simulink model "SRM_IOT"  (R2024b)
settings: Solver=VariableStepAuto  StartTime=0.0  StopTime=10.0  RelTol=1e-3
undefined symbols (not defined in the file): Ion, Lithium, sigbuilder_block
libraries: spsBreakerLib x120, spsSeriesRLCBranchLib x70, spsBatteryLib x42, spsIdealSwitchLib x33, spsVoltageMeasurementLib x27, slpidlib x17, spsMosfetLib x17, spsPWMGeneratorDCDCLib x11, spsDiodeLib x6, spsCurrentMeasurementLib x4, spsIGBTLib x2, spsThreePhaseSeriesRLCLoadLib x2
(part 3 of 5)

== system SRM_IOT/Subsystem18/Subsystem4 ==
  Battery : spsBatteryLib/Battery  BatType=Lithium-Ion  NomV=12  NomQ=10  SOC=95  Batt_Tr=30  PresetModel=on  MaxQ=10  MinV=9  FullV=13.9678  Dis_rate=4.3478  R=0.012  Normal_OP=9.0435  expZone="[12.9646     0.491304]"
  Breaker{,1..3} (4 alike) : spsBreakerLib/Breaker  InitialState=0  SwitchingTimes="[1/60  5/60]"  External=on  BreakerResistance=0.01  SnubberResistance=1e6  SnubberCapacitance=inf  Measurements=None  MoreParameters=on  NoBreakLoop=off
  Bus Selector : BusSelector  OutputSignals=SOC (%),Current (A),Voltage (V)
  Scope : Scope  NumInputPorts=3
  Series RLC Branch : spsSeriesRLCBranchLib/Series RLC Branch  LConnTagsString=__new0  RConnTagsString=__new0  BranchType=R  Resistance=1  Inductance=1e-3  SetiL0=off  InitialCurrent=0  Capacitance=1e-6  Setx0=off  InitialVoltage=0  Measurements=None
  + : PMIOPort  Side=Right
  - : PMIOPort  Port=2  Side=Right
  tag scope: s3=global
  wires:
  Battery/1 -> Bus Selector/1
  [c3] -> Breaker3/1, Breaker/1
  Bus Selector/2 -> Scope/2  "<Current (A)>"
  [d3] -> Breaker1/1, Breaker2/1
  Bus Selector/3 -> Scope/3  "<Voltage (V)>"
  Bus Selector/1 -> [s3], Scope/1  "<SOC (%)>"
  connections:
  Breaker2/LConn1 -- Breaker3/RConn1 -- Battery/LConn2
  Breaker1/LConn1 -- Battery/LConn1 -- Breaker/RConn1
  +/RConn1 -- Breaker/LConn1
  Series RLC Branch/LConn1 -- Breaker2/RConn1
  Series RLC Branch/RConn1 -- Breaker1/RConn1
  -/RConn1 -- Breaker3/LConn1

== system SRM_IOT/Subsystem18/Subsystem5 ==
  Battery : spsBatteryLib/Battery  BatType=Lithium-Ion  NomV=12  NomQ=10  SOC=95  Batt_Tr=30  PresetModel=on  MaxQ=10  MinV=9  FullV=13.9678  Dis_rate=4.3478  R=0.012  Normal_OP=9.0435  expZone="[12.9646     0.491304]"
  Breaker{,1..3} (4 alike) : spsBreakerLib/Breaker  InitialState=0  SwitchingTimes="[1/60  5/60]"  External=on  BreakerResistance=0.01  SnubberResistance=1e6  SnubberCapacitance=inf  Measurements=None  MoreParameters=on  NoBreakLoop=off
  Bus Selector : BusSelector  OutputSignals=SOC (%),Current (A),Voltage (V)
  Scope : Scope  NumInputPorts=3
  Series RLC Branch : spsSeriesRLCBranchLib/Series RLC Branch  LConnTagsString=__new0  RConnTagsString=__new0  BranchType=R  Resistance=1  Inductance=1e-3  SetiL0=off  InitialCurrent=0  Capacitance=1e-6  Setx0=off  InitialVoltage=0  Measurements=None
  + : PMIOPort  Side=Right
  - : PMIOPort  Port=2  Side=Right
  tag scope: s2=global
  wires:
  Battery/1 -> Bus Selector/1
  [c2] -> Breaker3/1, Breaker/1
  Bus Selector/2 -> Scope/2  "<Current (A)>"
  [d2] -> Breaker1/1, Breaker2/1
  Bus Selector/3 -> Scope/3  "<Voltage (V)>"
  Bus Selector/1 -> [s2], Scope/1  "<SOC (%)>"
  connections:
  Breaker2/LConn1 -- Breaker3/RConn1 -- Battery/LConn2
  Breaker1/LConn1 -- Battery/LConn1 -- Breaker/RConn1
  +/RConn1 -- Breaker/LConn1
  Series RLC Branch/LConn1 -- Breaker2/RConn1
  Series RLC Branch/RConn1 -- Breaker1/RConn1
  -/RConn1 -- Breaker3/LConn1

== system SRM_IOT/Subsystem18/Subsystem6 ==
  Battery : spsBatteryLib/Battery  BatType=Lithium-Ion  NomV=12  NomQ=10  SOC=95  Batt_Tr=30  PresetModel=on  MaxQ=10  MinV=9  FullV=13.9678  Dis_rate=4.3478  R=0.012  Normal_OP=9.0435  expZone="[12.9646     0.491304]"
  Breaker{,1..3} (4 alike) : spsBreakerLib/Breaker  InitialState=0  SwitchingTimes="[1/60  5/60]"  External=on  BreakerResistance=0.01  SnubberResistance=1e6  SnubberCapacitance=inf  Measurements=None  MoreParameters=on  NoBreakLoop=off
  Bus Selector : BusSelector  OutputSignals=SOC (%),Current (A),Voltage (V)
  Scope : Scope  NumInputPorts=3
  Series RLC Branch : spsSeriesRLCBranchLib/Series RLC Branch  LConnTagsString=__new0  RConnTagsString=__new0  BranchType=R  Resistance=1  Inductance=1e-3  SetiL0=off  InitialCurrent=0  Capacitance=1e-6  Setx0=off  InitialVoltage=0  Measurements=None
  + : PMIOPort  Side=Right
  - : PMIOPort  Port=2  Side=Right
  tag scope: s15=global
  wires:
  Battery/1 -> Bus Selector/1
  [c15] -> Breaker3/1, Breaker/1
  Bus Selector/2 -> Scope/2  "<Current (A)>"
  [d15] -> Breaker1/1, Breaker2/1
  Bus Selector/3 -> Scope/3  "<Voltage (V)>"
  Bus Selector/1 -> [s15], Scope/1  "<SOC (%)>"
  connections:
  Breaker2/LConn1 -- Breaker3/RConn1 -- Battery/LConn2
  Breaker1/LConn1 -- Battery/LConn1 -- Breaker/RConn1
  +/RConn1 -- Breaker/LConn1
  Series RLC Branch/LConn1 -- Breaker2/RConn1
  Series RLC Branch/RConn1 -- Breaker1/RConn1
  -/RConn1 -- Breaker3/LConn1

== system SRM_IOT/Subsystem18/Subsystem7 ==
  Battery : spsBatteryLib/Battery  BatType=Lithium-Ion  NomV=12  NomQ=10  SOC=95  Batt_Tr=30  PresetModel=on  MaxQ=10  MinV=9  FullV=13.9678  Dis_rate=4.3478  R=0.012  Normal_OP=9.0435  expZone="[12.9646     0.491304]"
  Breaker{,1..3} (4 alike) : spsBreakerLib/Breaker  InitialState=0  SwitchingTimes="[1/60  5/60]"  External=on  BreakerResistance=0.01  SnubberResistance=1e6  SnubberCapacitance=inf  Measurements=None  MoreParameters=on  NoBreakLoop=off
  Bus Selector : BusSelector  OutputSignals=SOC (%),Current (A),Voltage (V)
  Scope : Scope  NumInputPorts=3
  Series RLC Branch : spsSeriesRLCBranchLib/Series RLC Branch  LConnTagsString=__new0  RConnTagsString=__new0  BranchType=R  Resistance=1  Inductance=1e-3  SetiL0=off  InitialCurrent=0  Capacitance=1e-6  Setx0=off  InitialVoltage=0  Measurements=None
  + : PMIOPort  Side=Right
  - : PMIOPort  Port=2  Side=Right
  tag scope: s11=global
  wires:
  Battery/1 -> Bus Selector/1
  [c11] -> Breaker3/1, Breaker/1
  Bus Selector/2 -> Scope/2  "<Current (A)>"
  [d11] -> Breaker1/1, Breaker2/1
  Bus Selector/3 -> Scope/3  "<Voltage (V)>"
  Bus Selector/1 -> [s11], Scope/1  "<SOC (%)>"
  connections:
  Breaker2/LConn1 -- Breaker3/RConn1 -- Battery/LConn2
  Breaker1/LConn1 -- Battery/LConn1 -- Breaker/RConn1
  +/RConn1 -- Breaker/LConn1
  Series RLC Branch/LConn1 -- Breaker2/RConn1
  Series RLC Branch/RConn1 -- Breaker1/RConn1
  -/RConn1 -- Breaker3/LConn1

== system SRM_IOT/Subsystem18/Subsystem8 ==
  Battery : spsBatteryLib/Battery  BatType=Lithium-Ion  NomV=12  NomQ=10  SOC=95  Batt_Tr=30  PresetModel=on  MaxQ=10  MinV=9  FullV=13.9678  Dis_rate=4.3478  R=0.012  Normal_OP=9.0435  expZone="[12.9646     0.491304]"
  Breaker{,1..3} (4 alike) : spsBreakerLib/Breaker  InitialState=0  SwitchingTimes="[1/60  5/60]"  External=on  BreakerResistance=0.01  SnubberResistance=1e6  SnubberCapacitance=inf  Measurements=None  MoreParameters=on  NoBreakLoop=off
  Bus Selector : BusSelector  OutputSignals=SOC (%),Current (A),Voltage (V)
  Scope : Scope  NumInputPorts=3
  Series RLC Branch : spsSeriesRLCBranchLib/Series RLC Branch  LConnTagsString=__new0  RConnTagsString=__new0  BranchType=R  Resistance=1  Inductance=1e-3  SetiL0=off  InitialCurrent=0  Capacitance=1e-6  Setx0=off  InitialVoltage=0  Measurements=None
  + : PMIOPort  Side=Right
  - : PMIOPort  Port=2  Side=Right
  tag scope: s19=global
  wires:
  Battery/1 -> Bus Selector/1
  [c19] -> Breaker3/1, Breaker/1
  Bus Selector/2 -> Scope/2  "<Current (A)>"
  [d19] -> Breaker1/1, Breaker2/1
  Bus Selector/3 -> Scope/3  "<Voltage (V)>"
  Bus Selector/1 -> [s19], Scope/1  "<SOC (%)>"
  connections:
  Breaker2/LConn1 -- Breaker3/RConn1 -- Battery/LConn2
  Breaker1/LConn1 -- Battery/LConn1 -- Breaker/RConn1
  +/RConn1 -- Breaker/LConn1
  Series RLC Branch/LConn1 -- Breaker2/RConn1
  Series RLC Branch/RConn1 -- Breaker1/RConn1
  -/RConn1 -- Breaker3/LConn1

== system SRM_IOT/Subsystem18/Subsystem9 ==
  Battery : spsBatteryLib/Battery  BatType=Lithium-Ion  NomV=12  NomQ=10  SOC=95  Batt_Tr=30  PresetModel=on  MaxQ=10  MinV=9  FullV=13.9678  Dis_rate=4.3478  R=0.012  Normal_OP=9.0435  expZone="[12.9646     0.491304]"
  Breaker{,1..3} (4 alike) : spsBreakerLib/Breaker  InitialState=0  SwitchingTimes="[1/60  5/60]"  External=on  BreakerResistance=0.01  SnubberResistance=1e6  SnubberCapacitance=inf  Measurements=None  MoreParameters=on  NoBreakLoop=off
  Bus Selector : BusSelector  OutputSignals=SOC (%),Current (A),Voltage (V)
  Scope : Scope  NumInputPorts=3
  Series RLC Branch : spsSeriesRLCBranchLib/Series RLC Branch  LConnTagsString=__new0  RConnTagsString=__new0  BranchType=R  Resistance=1  Inductance=1e-3  SetiL0=off  InitialCurrent=0  Capacitance=1e-6  Setx0=off  InitialVoltage=0  Measurements=None
  + : PMIOPort  Side=Right
  - : PMIOPort  Port=2  Side=Right
  tag scope: s20=global
  wires:
  Battery/1 -> Bus Selector/1
  [c20] -> Breaker3/1, Breaker/1
  Bus Selector/2 -> Scope/2  "<Current (A)>"
  [d20] -> Breaker1/1, Breaker2/1
  Bus Selector/3 -> Scope/3  "<Voltage (V)>"
  Bus Selector/1 -> [s20], Scope/1  "<SOC (%)>"
  connections:
  Breaker2/LConn1 -- Breaker3/RConn1 -- Battery/LConn2
  Breaker1/LConn1 -- Battery/LConn1 -- Breaker/RConn1
  +/RConn1 -- Breaker/LConn1
  Series RLC Branch/LConn1 -- Breaker2/RConn1
  Series RLC Branch/RConn1 -- Breaker1/RConn1
  -/RConn1 -- Breaker3/LConn1

== system SRM_IOT/Subsystem2/Control ==
  Add : Sum  Inputs=+-
  Add1 : Sum  Inputs=+-
  Constant : Constant  Value=25.99
  Gain : Gain  Gain=-1
  NOT : Logic  Operator=NOT  IconShape=distinctive  AllPortsSameDT=off  OutDataTypeStr=boolean
  PID Controller : slpidlib/PID Controller  Controller=PI  Form=Parallel  TimeDomain=Continuous-time  UseExternalTs=off  SampleTime=-1  IntegratorMethod=Forward Euler  FilterMethod=Forward Euler  ControllerParametersSource=internal  P=0.005  I=10  UseKiTs=off  D=0  UseExternalDerivativeSource=off  N=100  UseFilter=on  TunerSelectOption=Transfer Function Based (PID Tuner App)  InitialConditionSource=internal  InitialConditionForIntegrator=0.54  InitialConditionForFilter=0  DifferentiatorICPrevScaledInput=0  ExternalReset=none  TrackingMode=off  Kt=1  LimitOutput=on  SatLimitsSource=internal  UpperSaturationLimit=0.975  LowerSaturationLimit=0  LinearizeAsGain=on  AntiWindupMode=none  Kb=1  LimitIntegrator=off  UpperIntegratorSaturationLimit=inf  LowerIntegratorSaturationLimit=-inf  POutMin=[]  POutMax=[]  IOutMin=[]  IOutMax=[]  DOutMin=[]  DOutMax=[]  NOutMin=[]  NOutMax=[]  SumOutMin=[]  SumOutMax=[]  SaturationOutMin=[]  SaturationOutMax=[]  PParamMin=[]  PParamMax=[]  IParamMin=[]  IParamMax=[]  DParamMin=[]  DParamMax=[]  NParamMin=[]  NParamMax=[]  KbParamMin=[]  KbParamMax=[]  KtParamMin=[]  KtParamMax=[]  KbOutMin=[]  KbOutMax=[]  KtOutMin=[]  KtOutMax=[]  IntegratorOutMin=[]  IntegratorOutMax=[]  FilterOutMin=[]  FilterOutMax=[]  SumI1OutMin=[]  SumI1OutMax=[]  SumI2OutMin=[]  SumI2OutMax=[]  SumI3OutMin=[]  SumI3OutMax=[]  SumI4OutMin=[]  SumI4OutMax=[]  SumDOutMin=[]  SumDOutMax=[]  DifferentiatorOutMin=[]  DifferentiatorOutMax=[]  FilterDiffOutCoefMin=[]  FilterDiffOutCoefMax=[]  ReciprocalOutMin=[]  ReciprocalOutMax=[]  SumDenOutMin=[]  SumDenOutMax=[]  SumNumOutMin=[]  SumNumOutMax=[]  DivideOutMin=[]  DivideOutMax=[]  UdiffTsProdOutMin=[]  UdiffTsProdOutMax=[]  NTsProdOutMin=[]  NTsProdOutMax=[]  UintegralTsProdOutMin=[]  UintegralTsProdOutMax=[]  UngainTsProdOutMin=[]  UngainTsProdOutMax=[]  ClampingZeroOutDataTypeStr=Inherit: Inherit via back propagation  ClampingZeroOutMin=[]  ClampingZeroOutMax=[]  FilterDenConstantOutDataTypeStr=Inherit: Inherit via back propagation  FilterDenConstantOutMin=[]  FilterDenConstantOutMax=[]  PCopyOutDataTypeStr=Inherit: Inherit via back propagation  PCopyOutMin=[]  PCopyOutMax=[]  NCopyOutDataTypeStr=Inherit: Inherit via back propagation  NCopyOutMin=[]  NCopyOutMax=[]  IntegratorContinuousStateAttributes=''  IntegratorStateMustResolveToSignalObject=off  IntegratorRTWStateStorageClass=Auto  FilterContinuousStateAttributes=''  FilterStateMustResolveToSignalObject=off  FilterRTWStateStorageClass=Auto  ParallelPVariant=InternalParameters  IdealPVariant=Disabled  IVariant=InternalParameters  DVariant=Disabled  IntegratorVariant=Continuous  SatVariant=Enabled  AWVariant=Passthrough  PCopyVariant=Disabled  TRVariant=Disabled  FdbkBlocksVariant=Forward  IdealPFdbkVariant=Disabled  SatFdbkVariant=Disabled  DerivativeFilterVariant=Disabled  NVariant=Disabled  NCopyVariant=Disabled_SignalSpec  FilterICVariant=Disabled  IntegratorICVariant=InternalICs  ExternalResetVariant=Disabled  TRSumVariant=Passthrough  SumFdbkVariant=Disabled  SumVariant=Sum_PI  TsampFilterVariant=InternalTs  TsampNgainVariant=Passthrough  TsampIntegralVariant=Disabled_SignalSpec  ExternalSaturationOutDataTypeStr=Inherit: Same as second input  DerivativeSourceVariant=Disabled  PreIntVariant=InternalPreInt
  PID Controller1 : slpidlib/PID Controller  Controller=PI  Form=Parallel  TimeDomain=Continuous-time  UseExternalTs=off  SampleTime=-1  IntegratorMethod=Forward Euler  FilterMethod=Forward Euler  ControllerParametersSource=internal  P=40  I=2000  UseKiTs=off  D=0  UseExternalDerivativeSource=off  N=100  UseFilter=on  TunerSelectOption=Transfer Function Based (PID Tuner App)  InitialConditionSource=internal  InitialConditionForIntegrator=0.54  InitialConditionForFilter=0  DifferentiatorICPrevScaledInput=0  ExternalReset=none  TrackingMode=off  Kt=1  LimitOutput=on  SatLimitsSource=internal  UpperSaturationLimit=17.39  LowerSaturationLimit=0  LinearizeAsGain=on  AntiWindupMode=none  Kb=1  LimitIntegrator=off  UpperIntegratorSaturationLimit=inf  LowerIntegratorSaturationLimit=-inf  POutMin=[]  POutMax=[]  IOutMin=[]  IOutMax=[]  DOutMin=[]  DOutMax=[]  NOutMin=[]  NOutMax=[]  SumOutMin=[]  SumOutMax=[]  SaturationOutMin=[]  SaturationOutMax=[]  PParamMin=[]  PParamMax=[]  IParamMin=[]  IParamMax=[]  DParamMin=[]  DParamMax=[]  NParamMin=[]  NParamMax=[]  KbParamMin=[]  KbParamMax=[]  KtParamMin=[]  KtParamMax=[]  KbOutMin=[]  KbOutMax=[]  KtOutMin=[]  KtOutMax=[]  IntegratorOutMin=[]  IntegratorOutMax=[]  FilterOutMin=[]  FilterOutMax=[]  SumI1OutMin=[]  SumI1OutMax=[]  SumI2OutMin=[]  SumI2OutMax=[]  SumI3OutMin=[]  SumI3OutMax=[]  SumI4OutMin=[]  SumI4OutMax=[]  SumDOutMin=[]  SumDOutMax=[]  DifferentiatorOutMin=[]  DifferentiatorOutMax=[]  FilterDiffOutCoefMin=[]  FilterDiffOutCoefMax=[]  ReciprocalOutMin=[]  ReciprocalOutMax=[]  SumDenOutMin=[]  SumDenOutMax=[]  SumNumOutMin=[]  SumNumOutMax=[]  DivideOutMin=[]  DivideOutMax=[]  UdiffTsProdOutMin=[]  UdiffTsProdOutMax=[]  NTsProdOutMin=[]  NTsProdOutMax=[]  UintegralTsProdOutMin=[]  UintegralTsProdOutMax=[]  UngainTsProdOutMin=[]  UngainTsProdOutMax=[]  ClampingZeroOutDataTypeStr=Inherit: Inherit via back propagation  ClampingZeroOutMin=[]  ClampingZeroOutMax=[]  FilterDenConstantOutDataTypeStr=Inherit: Inherit via back propagation  FilterDenConstantOutMin=[]  FilterDenConstantOutMax=[]  PCopyOutDataTypeStr=Inherit: Inherit via back propagation  PCopyOutMin=[]  PCopyOutMax=[]  NCopyOutDataTypeStr=Inherit: Inherit via back propagation  NCopyOutMin=[]  NCopyOutMax=[]  IntegratorContinuousStateAttributes=''  IntegratorStateMustResolveToSignalObject=off  IntegratorRTWStateStorageClass=Auto  FilterContinuousStateAttributes=''  FilterStateMustResolveToSignalObject=off  FilterRTWStateStorageClass=Auto  ParallelPVariant=InternalParameters  IdealPVariant=Disabled  IVariant=InternalParameters  DVariant=Disabled  IntegratorVariant=Continuous  SatVariant=Enabled  AWVariant=Passthrough  PCopyVariant=Disabled  TRVariant=Disabled  FdbkBlocksVariant=Forward  IdealPFdbkVariant=Disabled  SatFdbkVariant=Disabled  DerivativeFilterVariant=Disabled  NVariant=Disabled  NCopyVariant=Disabled_SignalSpec  FilterICVariant=Disabled  IntegratorICVariant=InternalICs  ExternalResetVariant=Disabled  TRSumVariant=Passthrough  SumFdbkVariant=Disabled  SumVariant=Sum_PI  TsampFilterVariant=InternalTs  TsampNgainVariant=Passthrough  TsampIntegralVariant=Disabled_SignalSpec  ExternalSaturationOutDataTypeStr=Inherit: Same as second input  DerivativeSourceVariant=Disabled  PreIntVariant=InternalPreInt
  PWM Generator (DC-DC) : spsPWMGeneratorDCDCLib/PWM Generator (DC-DC)  Fsw=10e3  Ts=5e-6
  tag scope: Mosfet_333=global, Mosfet_33=global
  wires:
  Add/1 -> PID Controller/1
  PWM Generator (DC-DC)/1 -> NOT/1, [Mosfet_33]
  PID Controller/1 -> PWM Generator (DC-DC)/1
  NOT/1 -> [Mosfet_333]
  [Ref_Current] -> Add/2
  [Current] -> Add/1
  PID Controller1/1 -> Gain/1
  Gain/1 -> [Ref_Current]
  Add1/1 -> PID Controller1/1
  Constant/1 -> Add1/1
  [Voltage] -> Add1/2

== system SRM_IOT/Subsystem3/Control ==
  Add : Sum  Inputs=+-
  Add1 : Sum  Inputs=+-
  Constant : Constant  Value=25.99
  Gain : Gain  Gain=-1
  NOT : Logic  Operator=NOT  IconShape=distinctive  AllPortsSameDT=off  OutDataTypeStr=boolean
  PID Controller : slpidlib/PID Controller  Controller=PI  Form=Parallel  TimeDomain=Continuous-time  UseExternalTs=off  SampleTime=-1  IntegratorMethod=Forward Euler  FilterMethod=Forward Euler  ControllerParametersSource=internal  P=0.005  I=10  UseKiTs=off  D=0  UseExternalDerivativeSource=off  N=100  UseFilter=on  TunerSelectOption=Transfer Function Based (PID Tuner App)  InitialConditionSource=internal  InitialConditionForIntegrator=0.54  InitialConditionForFilter=0  DifferentiatorICPrevScaledInput=0  ExternalReset=none  TrackingMode=off  Kt=1  LimitOutput=on  SatLimitsSource=internal  UpperSaturationLimit=0.975  LowerSaturationLimit=0  LinearizeAsGain=on  AntiWindupMode=none  Kb=1  LimitIntegrator=off  UpperIntegratorSaturationLimit=inf  LowerIntegratorSaturationLimit=-inf  POutMin=[]  POutMax=[]  IOutMin=[]  IOutMax=[]  DOutMin=[]  DOutMax=[]  NOutMin=[]  NOutMax=[]  SumOutMin=[]  SumOutMax=[]  SaturationOutMin=[]  SaturationOutMax=[]  PParamMin=[]  PParamMax=[]  IParamMin=[]  IParamMax=[]  DParamMin=[]  DParamMax=[]  NParamMin=[]  NParamMax=[]  KbParamMin=[]  KbParamMax=[]  KtParamMin=[]  KtParamMax=[]  KbOutMin=[]  KbOutMax=[]  KtOutMin=[]  KtOutMax=[]  IntegratorOutMin=[]  IntegratorOutMax=[]  FilterOutMin=[]  FilterOutMax=[]  SumI1OutMin=[]  SumI1OutMax=[]  SumI2OutMin=[]  SumI2OutMax=[]  SumI3OutMin=[]  SumI3OutMax=[]  SumI4OutMin=[]  SumI4OutMax=[]  SumDOutMin=[]  SumDOutMax=[]  DifferentiatorOutMin=[]  DifferentiatorOutMax=[]  FilterDiffOutCoefMin=[]  FilterDiffOutCoefMax=[]  ReciprocalOutMin=[]  ReciprocalOutMax=[]  SumDenOutMin=[]  SumDenOutMax=[]  SumNumOutMin=[]  SumNumOutMax=[]  DivideOutMin=[]  DivideOutMax=[]  UdiffTsProdOutMin=[]  UdiffTsProdOutMax=[]  NTsProdOutMin=[]  NTsProdOutMax=[]  UintegralTsProdOutMin=[]  UintegralTsProdOutMax=[]  UngainTsProdOutMin=[]  UngainTsProdOutMax=[]  ClampingZeroOutDataTypeStr=Inherit: Inherit via back propagation  ClampingZeroOutMin=[]  ClampingZeroOutMax=[]  FilterDenConstantOutDataTypeStr=Inherit: Inherit via back propagation  FilterDenConstantOutMin=[]  FilterDenConstantOutMax=[]  PCopyOutDataTypeStr=Inherit: Inherit via back propagation  PCopyOutMin=[]  PCopyOutMax=[]  NCopyOutDataTypeStr=Inherit: Inherit via back propagation  NCopyOutMin=[]  NCopyOutMax=[]  IntegratorContinuousStateAttributes=''  IntegratorStateMustResolveToSignalObject=off  IntegratorRTWStateStorageClass=Auto  FilterContinuousStateAttributes=''  FilterStateMustResolveToSignalObject=off  FilterRTWStateStorageClass=Auto  ParallelPVariant=InternalParameters  IdealPVariant=Disabled  IVariant=InternalParameters  DVariant=Disabled  IntegratorVariant=Continuous  SatVariant=Enabled  AWVariant=Passthrough  PCopyVariant=Disabled  TRVariant=Disabled  FdbkBlocksVariant=Forward  IdealPFdbkVariant=Disabled  SatFdbkVariant=Disabled  DerivativeFilterVariant=Disabled  NVariant=Disabled  NCopyVariant=Disabled_SignalSpec  FilterICVariant=Disabled  IntegratorICVariant=InternalICs  ExternalResetVariant=Disabled  TRSumVariant=Passthrough  SumFdbkVariant=Disabled  SumVariant=Sum_PI  TsampFilterVariant=InternalTs  TsampNgainVariant=Passthrough  TsampIntegralVariant=Disabled_SignalSpec  ExternalSaturationOutDataTypeStr=Inherit: Same as second input  DerivativeSourceVariant=Disabled  PreIntVariant=InternalPreInt
  PID Controller1 : slpidlib/PID Controller  Controller=PI  Form=Parallel  TimeDomain=Continuous-time  UseExternalTs=off  SampleTime=-1  IntegratorMethod=Forward Euler  FilterMethod=Forward Euler  ControllerParametersSource=internal  P=40  I=2000  UseKiTs=off  D=0  UseExternalDerivativeSource=off  N=100  UseFilter=on  TunerSelectOption=Transfer Function Based (PID Tuner App)  InitialConditionSource=internal  InitialConditionForIntegrator=0.54  InitialConditionForFilter=0  DifferentiatorICPrevScaledInput=0  ExternalReset=none  TrackingMode=off  Kt=1  LimitOutput=on  SatLimitsSource=internal  UpperSaturationLimit=17.39  LowerSaturationLimit=0  LinearizeAsGain=on  AntiWindupMode=none  Kb=1  LimitIntegrator=off  UpperIntegratorSaturationLimit=inf  LowerIntegratorSaturationLimit=-inf  POutMin=[]  POutMax=[]  IOutMin=[]  IOutMax=[]  DOutMin=[]  DOutMax=[]  NOutMin=[]  NOutMax=[]  SumOutMin=[]  SumOutMax=[]  SaturationOutMin=[]  SaturationOutMax=[]  PParamMin=[]  PParamMax=[]  IParamMin=[]  IParamMax=[]  DParamMin=[]  DParamMax=[]  NParamMin=[]  NParamMax=[]  KbParamMin=[]  KbParamMax=[]  KtParamMin=[]  KtParamMax=[]  KbOutMin=[]  KbOutMax=[]  KtOutMin=[]  KtOutMax=[]  IntegratorOutMin=[]  IntegratorOutMax=[]  FilterOutMin=[]  FilterOutMax=[]  SumI1OutMin=[]  SumI1OutMax=[]  SumI2OutMin=[]  SumI2OutMax=[]  SumI3OutMin=[]  SumI3OutMax=[]  SumI4OutMin=[]  SumI4OutMax=[]  SumDOutMin=[]  SumDOutMax=[]  DifferentiatorOutMin=[]  DifferentiatorOutMax=[]  FilterDiffOutCoefMin=[]  FilterDiffOutCoefMax=[]  ReciprocalOutMin=[]  ReciprocalOutMax=[]  SumDenOutMin=[]  SumDenOutMax=[]  SumNumOutMin=[]  SumNumOutMax=[]  DivideOutMin=[]  DivideOutMax=[]  UdiffTsProdOutMin=[]  UdiffTsProdOutMax=[]  NTsProdOutMin=[]  NTsProdOutMax=[]  UintegralTsProdOutMin=[]  UintegralTsProdOutMax=[]  UngainTsProdOutMin=[]  UngainTsProdOutMax=[]  ClampingZeroOutDataTypeStr=Inherit: Inherit via back propagation  ClampingZeroOutMin=[]  ClampingZeroOutMax=[]  FilterDenConstantOutDataTypeStr=Inherit: Inherit via back propagation  FilterDenConstantOutMin=[]  FilterDenConstantOutMax=[]  PCopyOutDataTypeStr=Inherit: Inherit via back propagation  PCopyOutMin=[]  PCopyOutMax=[]  NCopyOutDataTypeStr=Inherit: Inherit via back propagation  NCopyOutMin=[]  NCopyOutMax=[]  IntegratorContinuousStateAttributes=''  IntegratorStateMustResolveToSignalObject=off  IntegratorRTWStateStorageClass=Auto  FilterContinuousStateAttributes=''  FilterStateMustResolveToSignalObject=off  FilterRTWStateStorageClass=Auto  ParallelPVariant=InternalParameters  IdealPVariant=Disabled  IVariant=InternalParameters  DVariant=Disabled  IntegratorVariant=Continuous  SatVariant=Enabled  AWVariant=Passthrough  PCopyVariant=Disabled  TRVariant=Disabled  FdbkBlocksVariant=Forward  IdealPFdbkVariant=Disabled  SatFdbkVariant=Disabled  DerivativeFilterVariant=Disabled  NVariant=Disabled  NCopyVariant=Disabled_SignalSpec  FilterICVariant=Disabled  IntegratorICVariant=InternalICs  ExternalResetVariant=Disabled  TRSumVariant=Passthrough  SumFdbkVariant=Disabled  SumVariant=Sum_PI  TsampFilterVariant=InternalTs  TsampNgainVariant=Passthrough  TsampIntegralVariant=Disabled_SignalSpec  ExternalSaturationOutDataTypeStr=Inherit: Same as second input  DerivativeSourceVariant=Disabled  PreIntVariant=InternalPreInt
  PWM Generator (DC-DC) : spsPWMGeneratorDCDCLib/PWM Generator (DC-DC)  Fsw=10e3  Ts=5e-6
  tag scope: Mosfet_444=global, Mosfet_44=global
  wires:
  Add/1 -> PID Controller/1
  PWM Generator (DC-DC)/1 -> NOT/1, [Mosfet_44]
  PID Controller/1 -> PWM Generator (DC-DC)/1
  NOT/1 -> [Mosfet_444]
  [Ref_Current] -> Add/2
  [Current] -> Add/1
  PID Controller1/1 -> Gain/1
  Gain/1 -> [Ref_Current]
  Add1/1 -> PID Controller1/1
  Constant/1 -> Add1/1
  [Voltage] -> Add1/2

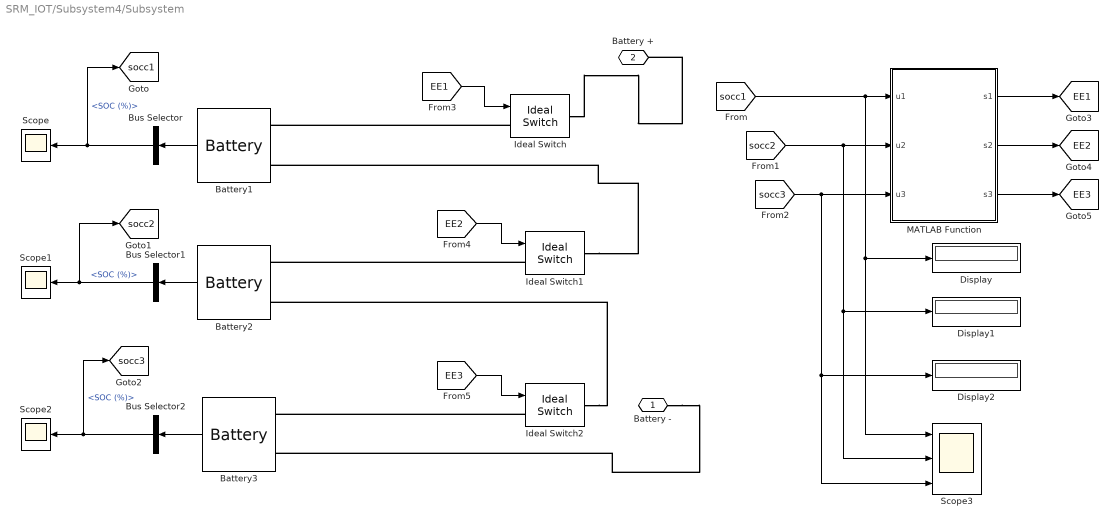
== system SRM_IOT/Subsystem4/Subsystem ==
  Battery1 : spsBatteryLib/Battery  BatType=Lithium-Ion  NomV=3.6  NomQ=4  SOC=100  Batt_Tr=1  PresetModel=on  MaxQ=4  MinV=2.7  FullV=4.1904  Dis_rate=1.7391  R=0.009  Normal_OP=3.6174  expZone="[3.8894     0.19652]"
  Battery2 : spsBatteryLib/Battery  BatType=Lithium-Ion  NomV=3.6  NomQ=4  SOC=60  Batt_Tr=1  PresetModel=on  MaxQ=4  MinV=2.7  FullV=4.1904  Dis_rate=1.7391  R=0.009  Normal_OP=3.6174  expZone="[3.8894     0.19652]"
  Battery3 : spsBatteryLib/Battery  BatType=Lithium-Ion  NomV=3.6  NomQ=4  SOC=30  Batt_Tr=1  PresetModel=on  MaxQ=4  MinV=2.7  FullV=4.1904  Dis_rate=1.7391  R=0.009  Normal_OP=3.6174  expZone="[3.8894     0.19652]"
  Bus Selector : BusSelector  OutputSignals=SOC (%)
  Bus Selector1 : BusSelector  OutputSignals=SOC (%)
  Bus Selector2 : BusSelector  OutputSignals=SOC (%)
  Display : Display
  Display1 : Display
  Display2 : Display
  Ideal Switch : spsIdealSwitchLib/Ideal Switch  Ron=0.001  Lon=0  IC=0  Rs=1e5  Cs=inf  Measurements=off
  Ideal Switch1 : spsIdealSwitchLib/Ideal Switch  Ron=0.001  Lon=0  IC=0  Rs=1e5  Cs=inf  Measurements=off
  Ideal Switch2 : spsIdealSwitchLib/Ideal Switch  Ron=0.001  Lon=0  IC=0  Rs=1e5  Cs=inf  Measurements=off
  MATLAB Function : MATLAB Function  TreatAsAtomicUnit=on
  Scope : Scope
  Scope1 : Scope
  Scope2 : Scope
  Scope3 : Scope  NumInputPorts=3
  Battery - : PMIOPort  Side=Left
  Battery + : PMIOPort  Port=2  Side=Left
  tag scope: EE1=global, EE2=global, EE3=global, socc1=global, socc2=global, socc3=global
  wires:
  Battery2/1 -> Bus Selector1/1
  Bus Selector/1 -> [socc1], Scope/1  "<SOC (%)>"
  [EE3] -> Ideal Switch2/1
  Bus Selector2/1 -> [socc3], Scope2/1  "<SOC (%)>"
  Bus Selector1/1 -> [socc2], Scope1/1  "<SOC (%)>"
  Battery3/1 -> Bus Selector2/1
  [socc2] -> MATLAB Function/2(u2), Display1/1, Scope3/2
  [socc1] -> Display/1, Scope3/1, MATLAB Function/1(u1)
  Battery1/1 -> Bus Selector/1
  [socc3] -> Display2/1, Scope3/3, MATLAB Function/3(u3)
  MATLAB Function/2(s2) -> [EE2]
  MATLAB Function/3(s3) -> [EE3]
  MATLAB Function/1(s1) -> [EE1]
  [EE1] -> Ideal Switch/1
  [EE2] -> Ideal Switch1/1
  connections:
  Ideal Switch1/RConn1 -- Battery1/LConn2
  Ideal Switch/RConn1 -- Battery +/RConn1
  Ideal Switch/LConn1 -- Battery1/LConn1
  Battery -/RConn1 -- Battery3/LConn2
  Ideal Switch2/RConn1 -- Battery2/LConn2
  Ideal Switch2/LConn1 -- Battery3/LConn1
  Ideal Switch1/LConn1 -- Battery2/LConn1

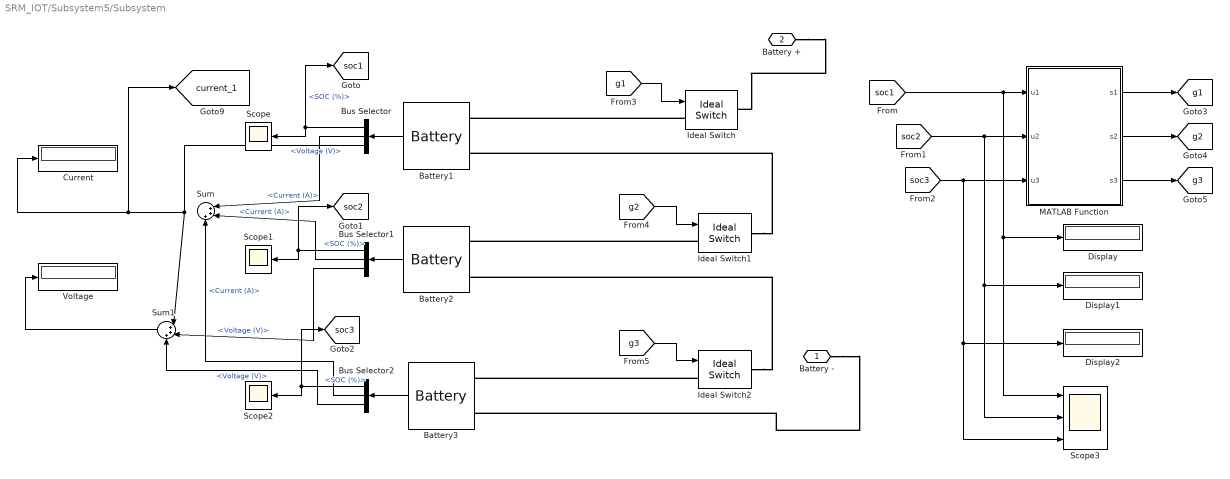
== system SRM_IOT/Subsystem5/Subsystem ==
  Battery1 : spsBatteryLib/Battery  BatType=Lithium-Ion  NomV=12  NomQ=100  SOC=100  Batt_Tr=1  PresetModel=on  MaxQ=100  MinV=9  FullV=13.9678  Dis_rate=43.4783  R=0.0012  Normal_OP=90.4348  expZone="[12.9646      4.91304]"
  Battery2 : spsBatteryLib/Battery  BatType=Lithium-Ion  NomV=12  NomQ=100  SOC=60  Batt_Tr=1  PresetModel=on  MaxQ=100  MinV=9  FullV=13.9678  Dis_rate=43.4783  R=0.0012  Normal_OP=90.4348  expZone="[12.9646      4.91304]"
  Battery3 : spsBatteryLib/Battery  BatType=Lithium-Ion  NomV=12  NomQ=100  SOC=30  Batt_Tr=1  PresetModel=on  MaxQ=100  MinV=9  FullV=13.9678  Dis_rate=43.4783  R=0.0012  Normal_OP=90.4348  expZone="[12.9646      4.91304]"
  Bus Selector : BusSelector  OutputSignals=SOC (%),Current (A),Voltage (V)
  Bus Selector1 : BusSelector  OutputSignals=SOC (%),Current (A),Voltage (V)
  Bus Selector2 : BusSelector  OutputSignals=SOC (%),Current (A),Voltage (V)
  Current : Display
  Display : Display
  Display1 : Display
  Display2 : Display
  Ideal Switch : spsIdealSwitchLib/Ideal Switch  Ron=0.001  Lon=0  IC=0  Rs=1e5  Cs=inf  Measurements=off
  Ideal Switch1 : spsIdealSwitchLib/Ideal Switch  Ron=0.001  Lon=0  IC=0  Rs=1e5  Cs=inf  Measurements=off
  Ideal Switch2 : spsIdealSwitchLib/Ideal Switch  Ron=0.001  Lon=0  IC=0  Rs=1e5  Cs=inf  Measurements=off
  MATLAB Function : MATLAB Function  TreatAsAtomicUnit=on
  Scope : Scope
  Scope1 : Scope
  Scope2 : Scope
  Scope3 : Scope  NumInputPorts=3
  Sum : Sum  Inputs=|+++
  Sum1 : Sum  Inputs=|+++
  Voltage : Display
  Battery - : PMIOPort  Side=Left
  Battery + : PMIOPort  Port=2  Side=Left
  tag scope: current_1=global, g1=global, g2=global, g3=global, soc1=global, soc2=global, soc3=global
  wires:
  Battery2/1 -> Bus Selector1/1
  Bus Selector/1 -> Scope/1, [soc1]  "<SOC (%)>"
  [g3] -> Ideal Switch2/1
  Bus Selector2/1 -> Scope2/1, [soc3]  "<SOC (%)>"
  Bus Selector1/1 -> Scope1/1, [soc2]  "<SOC (%)>"
  Battery3/1 -> Bus Selector2/1
  [soc2] -> MATLAB Function/2(u2), Display1/1, Scope3/2
  [soc1] -> Display/1, Scope3/1, MATLAB Function/1(u1)
  Battery1/1 -> Bus Selector/1
  [soc3] -> Display2/1, Scope3/3, MATLAB Function/3(u3)
  MATLAB Function/2(s2) -> [g2]
  MATLAB Function/3(s3) -> [g3]
  MATLAB Function/1(s1) -> [g1]
  [g1] -> Ideal Switch/1
  [g2] -> Ideal Switch1/1
  Bus Selector/2 -> Sum/1  "<Current (A)>"
  Bus Selector1/2 -> Sum/2  "<Current (A)>"
  Bus Selector2/2 -> Sum/3  "<Current (A)>"
  Bus Selector/3 -> [current_1], Current/1, Sum1/1  "<Voltage (V)>"
  Bus Selector1/3 -> Sum1/2  "<Voltage (V)>"
  Bus Selector2/3 -> Sum1/3  "<Voltage (V)>"
  Sum1/1 -> Voltage/1
  connections:
  Ideal Switch2/RConn1 -- Battery2/LConn2
  Battery +/RConn1 -- Ideal Switch/RConn1
  Ideal Switch2/LConn1 -- Battery3/LConn1
  Ideal Switch/LConn1 -- Battery1/LConn1
  Ideal Switch1/RConn1 -- Battery1/LConn2
  Ideal Switch1/LConn1 -- Battery2/LConn1
  Battery -/RConn1 -- Battery3/LConn2

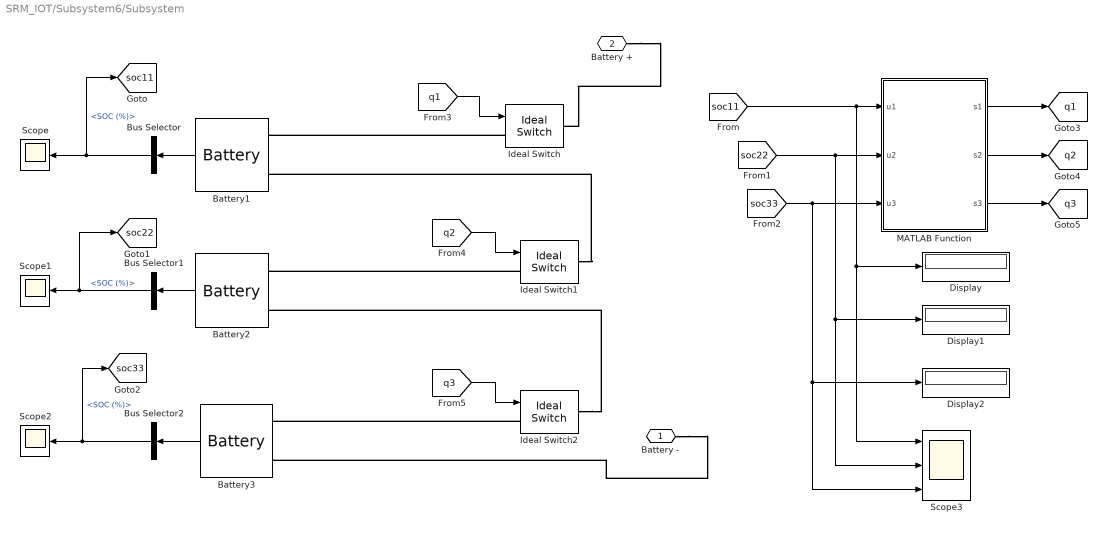
== system SRM_IOT/Subsystem6/Subsystem ==
  Battery1 : spsBatteryLib/Battery  BatType=Lithium-Ion  NomV=3.6  NomQ=4  SOC=100  Batt_Tr=1  PresetModel=on  MaxQ=4  MinV=2.7  FullV=4.1904  Dis_rate=1.7391  R=0.009  Normal_OP=3.6174  expZone="[3.8894     0.19652]"
  Battery2 : spsBatteryLib/Battery  BatType=Lithium-Ion  NomV=3.6  NomQ=4  SOC=60  Batt_Tr=1  PresetModel=on  MaxQ=4  MinV=2.7  FullV=4.1904  Dis_rate=1.7391  R=0.009  Normal_OP=3.6174  expZone="[3.8894     0.19652]"
  Battery3 : spsBatteryLib/Battery  BatType=Lithium-Ion  NomV=3.6  NomQ=4  SOC=30  Batt_Tr=1  PresetModel=on  MaxQ=4  MinV=2.7  FullV=4.1904  Dis_rate=1.7391  R=0.009  Normal_OP=3.6174  expZone="[3.8894     0.19652]"
  Bus Selector : BusSelector  OutputSignals=SOC (%)
  Bus Selector1 : BusSelector  OutputSignals=SOC (%)
  Bus Selector2 : BusSelector  OutputSignals=SOC (%)
  Display : Display
  Display1 : Display
  Display2 : Display
  Ideal Switch : spsIdealSwitchLib/Ideal Switch  Ron=0.001  Lon=0  IC=0  Rs=1e5  Cs=inf  Measurements=off
  Ideal Switch1 : spsIdealSwitchLib/Ideal Switch  Ron=0.001  Lon=0  IC=0  Rs=1e5  Cs=inf  Measurements=off
  Ideal Switch2 : spsIdealSwitchLib/Ideal Switch  Ron=0.001  Lon=0  IC=0  Rs=1e5  Cs=inf  Measurements=off
  MATLAB Function : MATLAB Function  TreatAsAtomicUnit=on
  Scope : Scope
  Scope1 : Scope
  Scope2 : Scope
  Scope3 : Scope  NumInputPorts=3
  Battery - : PMIOPort  Side=Left
  Battery + : PMIOPort  Port=2  Side=Left
  tag scope: q1=global, q2=global, q3=global, soc11=global, soc22=global, soc33=global
  wires:
  Battery2/1 -> Bus Selector1/1
  Bus Selector/1 -> [soc11], Scope/1  "<SOC (%)>"
  [q3] -> Ideal Switch2/1
  Bus Selector2/1 -> [soc33], Scope2/1  "<SOC (%)>"
  Bus Selector1/1 -> [soc22], Scope1/1  "<SOC (%)>"
  Battery3/1 -> Bus Selector2/1
  [soc22] -> MATLAB Function/2(u2), Display1/1, Scope3/2
  [soc11] -> Display/1, Scope3/1, MATLAB Function/1(u1)
  Battery1/1 -> Bus Selector/1
  [soc33] -> Display2/1, Scope3/3, MATLAB Function/3(u3)
  MATLAB Function/2(s2) -> [q2]
  MATLAB Function/3(s3) -> [q3]
  MATLAB Function/1(s1) -> [q1]
  [q1] -> Ideal Switch/1
  [q2] -> Ideal Switch1/1
  connections:
  Ideal Switch2/RConn1 -- Battery2/LConn2
  Battery +/RConn1 -- Ideal Switch/RConn1
  Ideal Switch1/LConn1 -- Battery2/LConn1
  Ideal Switch1/RConn1 -- Battery1/LConn2
  Battery -/RConn1 -- Battery3/LConn2
  Ideal Switch2/LConn1 -- Battery3/LConn1
  Ideal Switch/LConn1 -- Battery1/LConn1

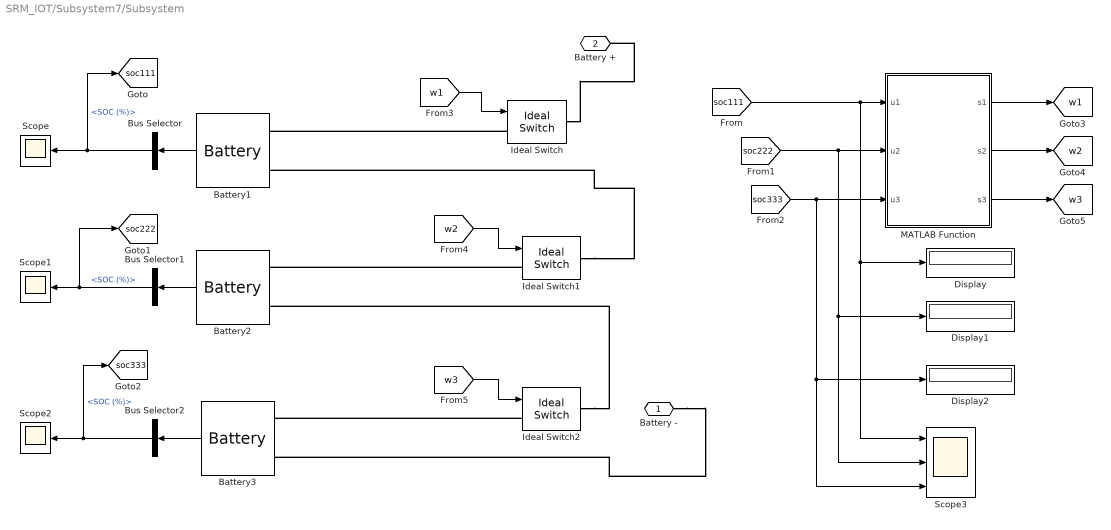
== system SRM_IOT/Subsystem7/Subsystem ==
  Battery1 : spsBatteryLib/Battery  BatType=Lithium-Ion  NomV=3.6  NomQ=4  SOC=100  Batt_Tr=1  PresetModel=on  MaxQ=4  MinV=2.7  FullV=4.1904  Dis_rate=1.7391  R=0.009  Normal_OP=3.6174  expZone="[3.8894     0.19652]"
  Battery2 : spsBatteryLib/Battery  BatType=Lithium-Ion  NomV=3.6  NomQ=4  SOC=60  Batt_Tr=1  PresetModel=on  MaxQ=4  MinV=2.7  FullV=4.1904  Dis_rate=1.7391  R=0.009  Normal_OP=3.6174  expZone="[3.8894     0.19652]"
  Battery3 : spsBatteryLib/Battery  BatType=Lithium-Ion  NomV=3.6  NomQ=4  SOC=30  Batt_Tr=1  PresetModel=on  MaxQ=4  MinV=2.7  FullV=4.1904  Dis_rate=1.7391  R=0.009  Normal_OP=3.6174  expZone="[3.8894     0.19652]"
  Bus Selector : BusSelector  OutputSignals=SOC (%)
  Bus Selector1 : BusSelector  OutputSignals=SOC (%)
  Bus Selector2 : BusSelector  OutputSignals=SOC (%)
  Display : Display
  Display1 : Display
  Display2 : Display
  Ideal Switch : spsIdealSwitchLib/Ideal Switch  Ron=0.001  Lon=0  IC=0  Rs=1e5  Cs=inf  Measurements=off
  Ideal Switch1 : spsIdealSwitchLib/Ideal Switch  Ron=0.001  Lon=0  IC=0  Rs=1e5  Cs=inf  Measurements=off
  Ideal Switch2 : spsIdealSwitchLib/Ideal Switch  Ron=0.001  Lon=0  IC=0  Rs=1e5  Cs=inf  Measurements=off
  MATLAB Function : MATLAB Function  TreatAsAtomicUnit=on
  Scope : Scope
  Scope1 : Scope
  Scope2 : Scope
  Scope3 : Scope  NumInputPorts=3
  Battery - : PMIOPort  Side=Left
  Battery + : PMIOPort  Port=2  Side=Left
  tag scope: soc111=global, soc222=global, soc333=global, w1=global, w2=global, w3=global
  wires:
  Battery2/1 -> Bus Selector1/1
  Bus Selector/1 -> [soc111], Scope/1  "<SOC (%)>"
  [w3] -> Ideal Switch2/1
  Bus Selector2/1 -> [soc333], Scope2/1  "<SOC (%)>"
  Bus Selector1/1 -> [soc222], Scope1/1  "<SOC (%)>"
  Battery3/1 -> Bus Selector2/1
  [soc222] -> MATLAB Function/2(u2), Display1/1, Scope3/2
  [soc111] -> Display/1, Scope3/1, MATLAB Function/1(u1)
  Battery1/1 -> Bus Selector/1
  [soc333] -> Display2/1, Scope3/3, MATLAB Function/3(u3)
  MATLAB Function/2(s2) -> [w2]
  MATLAB Function/3(s3) -> [w3]
  MATLAB Function/1(s1) -> [w1]
  [w1] -> Ideal Switch/1
  [w2] -> Ideal Switch1/1
  connections:
  Ideal Switch1/RConn1 -- Battery1/LConn2
  Ideal Switch/RConn1 -- Battery +/RConn1
  Ideal Switch/LConn1 -- Battery1/LConn1
  Battery -/RConn1 -- Battery3/LConn2
  Ideal Switch2/RConn1 -- Battery2/LConn2
  Ideal Switch2/LConn1 -- Battery3/LConn1
  Ideal Switch1/LConn1 -- Battery2/LConn1

== system SRM_IOT/Vechicle BMS Monitoring/BMS Discharge ==
  Terminal voltage : Inport
  Temperature : Inport  Port=2
  Current : Inport  Port=3
  Constant : Constant  Value=0
  Function logic block : Subsystem
  Switch : Switch  Criteria=u2 ~= 0  SaturateOnIntegerOverflow=off  InputSameDT=off
  Discharge current : Outport
  wires:
  Terminal voltage/1 -> Function logic block/1(Terminal voltage)
  Current/1 -> Switch/3, Function logic block/2(Current)
  Temperature/1 -> Function logic block/3(Temperature)
  Function logic block/1(Discharge Terget) -> Switch/2
  Constant/1 -> Switch/1
  Switch/1 -> Discharge current/1

== system SRM_IOT/Vechicle BMS Monitoring1/BMS Discharge ==
  Terminal voltage : Inport
  Temperature : Inport  Port=2
  Current : Inport  Port=3
  Constant : Constant  Value=0
  Function logic block : Subsystem
  Switch : Switch  Criteria=u2 ~= 0  SaturateOnIntegerOverflow=off  InputSameDT=off
  Discharge current : Outport
  wires:
  Terminal voltage/1 -> Function logic block/1(Terminal voltage)
  Current/1 -> Switch/3, Function logic block/2(Current)
  Temperature/1 -> Function logic block/3(Temperature)
  Function logic block/1(Discharge Terget) -> Switch/2
  Constant/1 -> Switch/1
  Switch/1 -> Discharge current/1

== system SRM_IOT/Vechicle BMS Monitoring2/BMS Discharge ==
  Terminal voltage : Inport
  Temperature : Inport  Port=2
  Current : Inport  Port=3
  Constant : Constant  Value=0
  Function logic block : Subsystem
  Switch : Switch  Criteria=u2 ~= 0  SaturateOnIntegerOverflow=off  InputSameDT=off
  Discharge current : Outport
  wires:
  Terminal voltage/1 -> Function logic block/1(Terminal voltage)
  Current/1 -> Switch/3, Function logic block/2(Current)
  Temperature/1 -> Function logic block/3(Temperature)
  Function logic block/1(Discharge Terget) -> Switch/2
  Constant/1 -> Switch/1
  Switch/1 -> Discharge current/1

== system SRM_IOT/Vechicle BMS Monitoring3/BMS Discharge ==
  Terminal voltage : Inport
  Temperature : Inport  Port=2
  Current : Inport  Port=3
  Constant : Constant  Value=0
  Function logic block : Subsystem
  Switch : Switch  Criteria=u2 ~= 0  SaturateOnIntegerOverflow=off  InputSameDT=off
  Discharge current : Outport
  wires:
  Terminal voltage/1 -> Function logic block/1(Terminal voltage)
  Current/1 -> Switch/3, Function logic block/2(Current)
  Temperature/1 -> Function logic block/3(Temperature)
  Function logic block/1(Discharge Terget) -> Switch/2
  Constant/1 -> Switch/1
  Switch/1 -> Discharge current/1

== system SRM_IOT/Fast charging controller/Fast charging Switching controller/g1 ==
  Constant1 : Constant  Value=0
  Constant2 : Constant
  Display2 : Display
  Display3 : Display
  Switch : Switch  Threshold=150  SaturateOnIntegerOverflow=off  InputSameDT=off
  tag scope: gg1=global
  wires:
  [FS] -> Display3/1, Switch/2
  Switch/1 -> Display2/1, [gg1]
  Constant1/1 -> Switch/3
  Constant2/1 -> Switch/1

== system SRM_IOT/Fast charging controller/Fast charging Switching controller/g2 ==
  Constant1 : Constant  Value=0
  Constant2 : Constant
  Display2 : Display
  Display3 : Display
  Switch : Switch  Threshold=150  SaturateOnIntegerOverflow=off  InputSameDT=off
  tag scope: gg2=global
  wires:
  [FS] -> Display3/1, Switch/2
  Switch/1 -> Display2/1, [gg2]
  Constant1/1 -> Switch/3
  Constant2/1 -> Switch/1

== system SRM_IOT/Fast charging controller/Fast charging Switching controller/g3 ==
  Constant1 : Constant  Value=0
  Constant2 : Constant
  Display2 : Display
  Display3 : Display
  Switch : Switch  Threshold=150  SaturateOnIntegerOverflow=off  InputSameDT=off
  tag scope: gg3=global
  wires:
  [FS] -> Display3/1, Switch/2
  Switch/1 -> Display2/1, [gg3]
  Constant1/1 -> Switch/3
  Constant2/1 -> Switch/1

== system SRM_IOT/Fast charging controller/Fast charging Switching controller/g4 ==
  Constant1 : Constant  Value=0
  Constant2 : Constant
  Display2 : Display
  Display3 : Display
  Switch : Switch  Threshold=150  SaturateOnIntegerOverflow=off  InputSameDT=off
  tag scope: gg4=global
  wires:
  [FS] -> Display3/1, Switch/2
  Switch/1 -> Display2/1, [gg4]
  Constant1/1 -> Switch/3
  Constant2/1 -> Switch/1

== system SRM_IOT/Grid/Wall charger Connection Box/Battery Switching Control ==
  Control : Inport
  Ideal Switch{,1,3..4} (4 alike) : spsIdealSwitchLib/Ideal Switch  Ron=0.001  Lon=0  IC=0  Rs=1e5  Cs=inf  Measurements=off
  NOT : Logic  Operator=NOT  IconShape=distinctive  AllPortsSameDT=off  OutDataTypeStr=boolean
  discharge + : PMIOPort  Side=Left
  discharge - : PMIOPort  Port=2  Side=Left
  charge + : PMIOPort  Port=3  Side=Left
  charge - : PMIOPort  Port=4  Side=Left
  battery + : PMIOPort  Port=5  Side=Right
  battery - : PMIOPort  Port=6  Side=Right
  wires:
  Control/1 -> NOT/1, Ideal Switch1/1, Ideal Switch/1
  NOT/1 -> Ideal Switch4/1, Ideal Switch3/1
  connections:
  charge -/RConn1 -- Ideal Switch4/RConn1
  discharge +/RConn1 -- Ideal Switch/RConn1
  Ideal Switch1/LConn1 -- battery -/RConn1 -- Ideal Switch4/LConn1
  discharge -/RConn1 -- Ideal Switch1/RConn1
  Ideal Switch/LConn1 -- battery +/RConn1 -- Ideal Switch3/LConn1
  charge +/RConn1 -- Ideal Switch3/RConn1

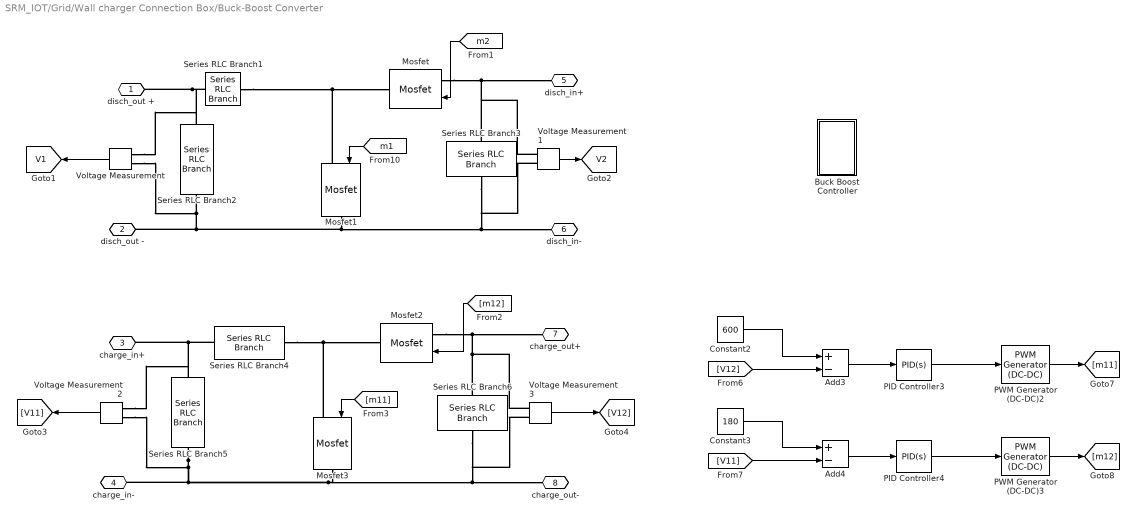
== system SRM_IOT/Grid/Wall charger Connection Box/Buck-Boost Converter ==
  Add3 : Sum  Inputs=+-
  Add4 : Sum  Inputs=+-
  Buck Boost Controller : Subsystem
  Constant2 : Constant  Value=600
  Constant3 : Constant  Value=180
  Mosfet{,1..3} (4 alike) : spsMosfetLib/Mosfet  Ron=0.1  Lon=0  Rd=0.01  Vfd=0  IC=0  Rs=1e5  Cs=inf  Measurements=off
  PID Controller3 : slpidlib/PID Controller  Controller=PID  Form=Parallel  TimeDomain=Continuous-time  UseExternalTs=off  SampleTime=-1  IntegratorMethod=Forward Euler  FilterMethod=Forward Euler  ControllerParametersSource=internal  P=0  I=7  UseKiTs=off  D=0  UseExternalDerivativeSource=off  N=100  UseFilter=on  TunerSelectOption=Transfer Function Based (PID Tuner App)  InitialConditionSource=internal  InitialConditionForIntegrator=0  InitialConditionForFilter=0  DifferentiatorICPrevScaledInput=0  ExternalReset=none  TrackingMode=off  Kt=1  LimitOutput=off  SatLimitsSource=internal  UpperSaturationLimit=inf  LowerSaturationLimit=-inf  LinearizeAsGain=on  AntiWindupMode=none  Kb=1  LimitIntegrator=off  UpperIntegratorSaturationLimit=inf  LowerIntegratorSaturationLimit=-inf  POutMin=[]  POutMax=[]  IOutMin=[]  IOutMax=[]  DOutMin=[]  DOutMax=[]  NOutMin=[]  NOutMax=[]  SumOutMin=[]  SumOutMax=[]  SaturationOutMin=[]  SaturationOutMax=[]  PParamMin=[]  PParamMax=[]  IParamMin=[]  IParamMax=[]  DParamMin=[]  DParamMax=[]  NParamMin=[]  NParamMax=[]  KbParamMin=[]  KbParamMax=[]  KtParamMin=[]  KtParamMax=[]  KbOutMin=[]  KbOutMax=[]  KtOutMin=[]  KtOutMax=[]  IntegratorOutMin=[]  IntegratorOutMax=[]  FilterOutMin=[]  FilterOutMax=[]  SumI1OutMin=[]  SumI1OutMax=[]  SumI2OutMin=[]  SumI2OutMax=[]  SumI3OutMin=[]  SumI3OutMax=[]  SumI4OutMin=[]  SumI4OutMax=[]  SumDOutMin=[]  SumDOutMax=[]  DifferentiatorOutMin=[]  DifferentiatorOutMax=[]  FilterDiffOutCoefMin=[]  FilterDiffOutCoefMax=[]  ReciprocalOutMin=[]  ReciprocalOutMax=[]  SumDenOutMin=[]  SumDenOutMax=[]  SumNumOutMin=[]  SumNumOutMax=[]  DivideOutMin=[]  DivideOutMax=[]  UdiffTsProdOutMin=[]  UdiffTsProdOutMax=[]  NTsProdOutMin=[]  NTsProdOutMax=[]  UintegralTsProdOutMin=[]  UintegralTsProdOutMax=[]  UngainTsProdOutMin=[]  UngainTsProdOutMax=[]  ClampingZeroOutDataTypeStr=Inherit: Inherit via back propagation  ClampingZeroOutMin=[]  ClampingZeroOutMax=[]  FilterDenConstantOutDataTypeStr=Inherit: Inherit via back propagation  FilterDenConstantOutMin=[]  FilterDenConstantOutMax=[]  PCopyOutDataTypeStr=Inherit: Inherit via back propagation  PCopyOutMin=[]  PCopyOutMax=[]  NCopyOutDataTypeStr=Inherit: Inherit via back propagation  NCopyOutMin=[]  NCopyOutMax=[]  IntegratorContinuousStateAttributes=''  IntegratorStateMustResolveToSignalObject=off  IntegratorRTWStateStorageClass=Auto  FilterContinuousStateAttributes=''  FilterStateMustResolveToSignalObject=off  FilterRTWStateStorageClass=Auto  ParallelPVariant=InternalParameters  IdealPVariant=Disabled  IVariant=InternalParameters  DVariant=InternalParameters  IntegratorVariant=Continuous  SatVariant=Disabled  AWVariant=Passthrough  PCopyVariant=Disabled  TRVariant=Disabled  FdbkBlocksVariant=Forward  IdealPFdbkVariant=Disabled  SatFdbkVariant=Disabled  DerivativeFilterVariant=ContFilter  NVariant=InternalParameters  NCopyVariant=Disabled  FilterICVariant=InternalICsFilter  IntegratorICVariant=InternalICs  ExternalResetVariant=Disabled  TRSumVariant=Passthrough  SumFdbkVariant=Disabled  SumVariant=Sum_PID  TsampFilterVariant=InternalTs  TsampNgainVariant=Passthrough  TsampIntegralVariant=Disabled_SignalSpec  ExternalSaturationOutDataTypeStr=Inherit: Same as second input  DerivativeSourceVariant=ErrorSignal  PreIntVariant=InternalPreInt
  PID Controller4 : slpidlib/PID Controller  Controller=PID  Form=Parallel  TimeDomain=Continuous-time  UseExternalTs=off  SampleTime=-1  IntegratorMethod=Forward Euler  FilterMethod=Forward Euler  ControllerParametersSource=internal  P=0  I=7  UseKiTs=off  D=0  UseExternalDerivativeSource=off  N=100  UseFilter=on  TunerSelectOption=Transfer Function Based (PID Tuner App)  InitialConditionSource=internal  InitialConditionForIntegrator=0  InitialConditionForFilter=0  DifferentiatorICPrevScaledInput=0  ExternalReset=none  TrackingMode=off  Kt=1  LimitOutput=off  SatLimitsSource=internal  UpperSaturationLimit=inf  LowerSaturationLimit=-inf  LinearizeAsGain=on  AntiWindupMode=none  Kb=1  LimitIntegrator=off  UpperIntegratorSaturationLimit=inf  LowerIntegratorSaturationLimit=-inf  POutMin=[]  POutMax=[]  IOutMin=[]  IOutMax=[]  DOutMin=[]  DOutMax=[]  NOutMin=[]  NOutMax=[]  SumOutMin=[]  SumOutMax=[]  SaturationOutMin=[]  SaturationOutMax=[]  PParamMin=[]  PParamMax=[]  IParamMin=[]  IParamMax=[]  DParamMin=[]  DParamMax=[]  NParamMin=[]  NParamMax=[]  KbParamMin=[]  KbParamMax=[]  KtParamMin=[]  KtParamMax=[]  KbOutMin=[]  KbOutMax=[]  KtOutMin=[]  KtOutMax=[]  IntegratorOutMin=[]  IntegratorOutMax=[]  FilterOutMin=[]  FilterOutMax=[]  SumI1OutMin=[]  SumI1OutMax=[]  SumI2OutMin=[]  SumI2OutMax=[]  SumI3OutMin=[]  SumI3OutMax=[]  SumI4OutMin=[]  SumI4OutMax=[]  SumDOutMin=[]  SumDOutMax=[]  DifferentiatorOutMin=[]  DifferentiatorOutMax=[]  FilterDiffOutCoefMin=[]  FilterDiffOutCoefMax=[]  ReciprocalOutMin=[]  ReciprocalOutMax=[]  SumDenOutMin=[]  SumDenOutMax=[]  SumNumOutMin=[]  SumNumOutMax=[]  DivideOutMin=[]  DivideOutMax=[]  UdiffTsProdOutMin=[]  UdiffTsProdOutMax=[]  NTsProdOutMin=[]  NTsProdOutMax=[]  UintegralTsProdOutMin=[]  UintegralTsProdOutMax=[]  UngainTsProdOutMin=[]  UngainTsProdOutMax=[]  ClampingZeroOutDataTypeStr=Inherit: Inherit via back propagation  ClampingZeroOutMin=[]  ClampingZeroOutMax=[]  FilterDenConstantOutDataTypeStr=Inherit: Inherit via back propagation  FilterDenConstantOutMin=[]  FilterDenConstantOutMax=[]  PCopyOutDataTypeStr=Inherit: Inherit via back propagation  PCopyOutMin=[]  PCopyOutMax=[]  NCopyOutDataTypeStr=Inherit: Inherit via back propagation  NCopyOutMin=[]  NCopyOutMax=[]  IntegratorContinuousStateAttributes=''  IntegratorStateMustResolveToSignalObject=off  IntegratorRTWStateStorageClass=Auto  FilterContinuousStateAttributes=''  FilterStateMustResolveToSignalObject=off  FilterRTWStateStorageClass=Auto  ParallelPVariant=InternalParameters  IdealPVariant=Disabled  IVariant=InternalParameters  DVariant=InternalParameters  IntegratorVariant=Continuous  SatVariant=Disabled  AWVariant=Passthrough  PCopyVariant=Disabled  TRVariant=Disabled  FdbkBlocksVariant=Forward  IdealPFdbkVariant=Disabled  SatFdbkVariant=Disabled  DerivativeFilterVariant=ContFilter  NVariant=InternalParameters  NCopyVariant=Disabled  FilterICVariant=InternalICsFilter  IntegratorICVariant=InternalICs  ExternalResetVariant=Disabled  TRSumVariant=Passthrough  SumFdbkVariant=Disabled  SumVariant=Sum_PID  TsampFilterVariant=InternalTs  TsampNgainVariant=Passthrough  TsampIntegralVariant=Disabled_SignalSpec  ExternalSaturationOutDataTypeStr=Inherit: Same as second input  DerivativeSourceVariant=ErrorSignal  PreIntVariant=InternalPreInt
  PWM Generator (DC-DC)2 : spsPWMGeneratorDCDCLib/PWM Generator (DC-DC)  Fsw=5000  Ts=0
  PWM Generator (DC-DC)3 : spsPWMGeneratorDCDCLib/PWM Generator (DC-DC)  Fsw=5000  Ts=0
  Series RLC Branch1 : spsSeriesRLCBranchLib/Series RLC Branch  LConnTagsString=__new0  RConnTagsString=__new0  BranchType=L  Resistance=1  Inductance=1e-3  SetiL0=off  InitialCurrent=0  Capacitance=1e-6  Setx0=off  InitialVoltage=0  Measurements=None
  Series RLC Branch{2..3,5..6} (4 alike) : spsSeriesRLCBranchLib/Series RLC Branch  LConnTagsString=__new0  RConnTagsString=__new0  BranchType=RC  Resistance=0.0001  Inductance=1e-3  SetiL0=off  InitialCurrent=0  Capacitance=1000e-6  Setx0=off  InitialVoltage=0  Measurements=None
  Series RLC Branch4 : spsSeriesRLCBranchLib/Series RLC Branch  LConnTagsString=__new0  RConnTagsString=__new0  BranchType=L  Resistance=100e3  Inductance=1e-3  SetiL0=off  InitialCurrent=0  Capacitance=1e-6  Setx0=off  InitialVoltage=0  Measurements=None
  Voltage Measurement{,1..3} (4 alike) : spsVoltageMeasurementLib/Voltage Measurement  PhasorSimulation=off  OutputType=Complex  PSBequivalent=0
  disch_out + : PMIOPort  Side=Left
  disch_out - : PMIOPort  Port=2  Side=Left
  charge_in+ : PMIOPort  Port=3  Side=Left
  charge_in- : PMIOPort  Port=4  Side=Left
  disch_in+ : PMIOPort  Port=5  Side=Right
  disch_in- : PMIOPort  Port=6  Side=Right
  charge_out+ : PMIOPort  Port=7  Side=Right
  charge_out- : PMIOPort  Port=8  Side=Right
  tag scope: V1=global, V2=global
  wires:
  Voltage Measurement1/1 -> [V2]
  Voltage Measurement/1 -> [V1]
  PWM Generator (DC-DC)2/1 -> [m11]
  [V11] -> Add4/2
  Add3/1 -> PID Controller3/1
  Voltage Measurement3/1 -> [V12]
  PID Controller4/1 -> PWM Generator (DC-DC)3/1
  PID Controller3/1 -> PWM Generator (DC-DC)2/1
  Add4/1 -> PID Controller4/1
  [m11] -> Mosfet3/1
  Voltage Measurement2/1 -> [V11]
  PWM Generator (DC-DC)3/1 -> [m12]
  [m12] -> Mosfet2/1
  Constant3/1 -> Add4/1
  Constant2/1 -> Add3/1
  [V12] -> Add3/2
  [m1] -> Mosfet1/1
  [m2] -> Mosfet/1
  connections:
  Series RLC Branch5/RConn1 -- charge_in-/RConn1 -- charge_out-/RConn1 -- Voltage Measurement3/LConn2 -- Series RLC Branch6/RConn1 -- Mosfet3/RConn1 -- Voltage Measurement2/LConn2
  Mosfet1/RConn1 -- disch_in-/RConn1 -- Voltage Measurement1/LConn2 -- Series RLC Branch3/RConn1 -- disch_out -/RConn1 -- Voltage Measurement/LConn2 -- Series RLC Branch2/RConn1
  Mosfet/LConn1 -- disch_in+/RConn1 -- Voltage Measurement1/LConn1 -- Series RLC Branch3/LConn1
  Series RLC Branch4/LConn1 -- charge_in+/RConn1 -- Voltage Measurement2/LConn1 -- Series RLC Branch5/LConn1
  Series RLC Branch1/LConn1 -- Voltage Measurement/LConn1 -- Series RLC Branch2/LConn1 -- disch_out +/RConn1
  Series RLC Branch6/LConn1 -- Voltage Measurement3/LConn1 -- charge_out+/RConn1 -- Mosfet2/LConn1
  Mosfet1/LConn1 -- Series RLC Branch1/RConn1 -- Mosfet/RConn1
  Series RLC Branch4/RConn1 -- Mosfet3/LConn1 -- Mosfet2/RConn1

== system SRM_IOT/Grid/Wall charger Connection Box/Connection Control ==
  Control : Inport
  Ideal Switch{,1..5} (6 alike) : spsIdealSwitchLib/Ideal Switch  Ron=0.001  Lon=0  IC=0  Rs=1e5  Cs=inf  Measurements=off
  NOT : Logic  Operator=NOT  IconShape=distinctive  AllPortsSameDT=off  OutDataTypeStr=boolean
  Grid R : PMIOPort  Side=Left
  Grid Y : PMIOPort  Port=2  Side=Left
  Grid B : PMIOPort  Port=3  Side=Left
  Discharge R : PMIOPort  Port=4  Side=Right
  Discharge Y : PMIOPort  Port=5  Side=Right
  Discharge B : PMIOPort  Port=6  Side=Right
  charge R : PMIOPort  Port=7  Side=Right
  charge Y : PMIOPort  Port=8  Side=Right
  charge B : PMIOPort  Port=9  Side=Right
  wires:
  Control/1 -> NOT/1, Ideal Switch2/1, Ideal Switch1/1, Ideal Switch/1
  NOT/1 -> Ideal Switch5/1, Ideal Switch4/1, Ideal Switch3/1
  connections:
  Ideal Switch2/RConn1 -- Grid B/RConn1 -- Ideal Switch5/RConn1
  Discharge R/RConn1 -- Ideal Switch/LConn1
  Discharge B/RConn1 -- Ideal Switch2/LConn1
  Ideal Switch/RConn1 -- Grid R/RConn1 -- Ideal Switch3/RConn1
  Ideal Switch1/RConn1 -- Grid Y/RConn1 -- Ideal Switch4/RConn1
  Ideal Switch4/LConn1 -- charge Y/RConn1
  Discharge Y/RConn1 -- Ideal Switch1/LConn1
  charge R/RConn1 -- Ideal Switch3/LConn1
  Ideal Switch5/LConn1 -- charge B/RConn1
